simulink model "model1"  (R2024a)
settings: Solver=VariableStepAuto  StartTime=0.0  StopTime=10.0  MaxStep=1e-4  RelTol=1e-3
values from neighbouring files (symbols this model uses):
  a0 = -2    [script11.m]    (also in script12.m)
  a1 = 1    [script11.m]    (also in script12.m)
  a2 = 1    [script11.m]    (also in script12.m)
  k0 = -15    [script12.m]
  k1 = -1.5    [script12.m]
settings Model: Creator=eva  LastModifiedBy=eva

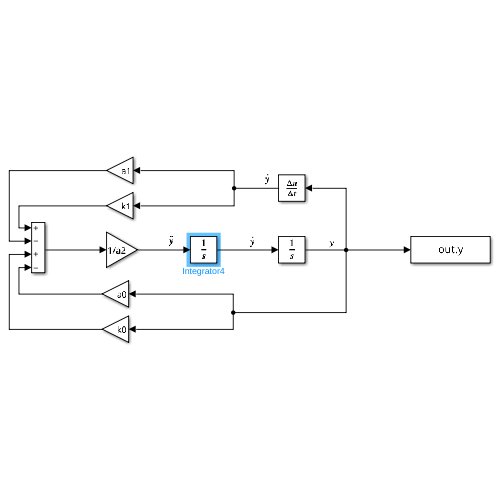
[thumbnail: Simulink's stored preview of the top-level diagram]
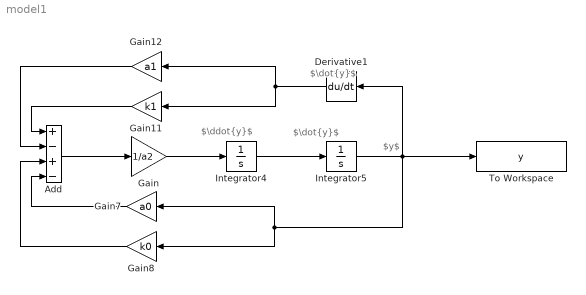
== system model1 ==
  note: $\dot{y}$
  note: $y$
  note: $\dot{y}$
  note: $\ddot{y}$
  Add : Sum  Inputs=+-+-
  Derivative1 : Derivative
  Gain : Gain  Gain=1/a2
  Gain11 : Gain  Gain=k1
  Gain12 : Gain  Gain=a1
  Gain7 : Gain  Gain=a0
  Gain8 : Gain  Gain=k0
  Integrator4 : Integrator  InitialCondition=-1
  Integrator5 : Integrator
  To Workspace : ToWorkspace  VariableName=y  SaveFormat=Structure With Time  SampleTime=-1
  wires:
  Integrator4/1 -> Integrator5/1
  Derivative1/1 -> Gain12/1, Gain11/1
  Integrator5/1 -> To Workspace/1, Derivative1/1, Gain7/1, Gain8/1
  Gain12/1 -> Add/2
  Gain11/1 -> Add/1
  Gain8/1 -> Add/3
  Gain7/1 -> Add/4
  Add/1 -> Gain/1
  Gain/1 -> Integrator4/1
